simulink model "sim_kalman03_p_u"  (R2015a)
settings: Solver=ode45  StartTime=1  StopTime=100  MaxStep=1  MinStep=1  RelTol=1e-8
undefined symbols (not defined in the file or in its folder): Discrete, Time
libraries: ctrlSharedLib x1
settings Model: Creator=liuqi  LastModifiedBy=liuqi
settings SolverCC: InitialStep=1

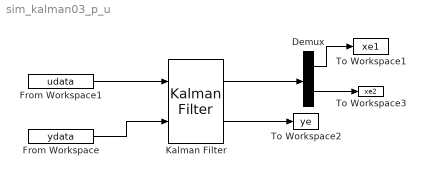
== system sim_kalman03_p_u ==
  Demux : Demux  Outputs=2
  From Workspace : FromWorkspace  VariableName=ydata  SampleTime=1  Interpolate=off  OutputAfterFinalValue=Setting to zero
  From Workspace1 : FromWorkspace  VariableName=udata  SampleTime=1  Interpolate=off  OutputAfterFinalValue=Setting to zero
  Kalman Filter : ctrlSharedLib/Kalman Filter  TimeDomain=Discrete-Time  UseCurrentEstimator=on  ModelSource=Individual A, B, C, D matrices  ModelSourceVariable=sys  A=[1,1;0,1]  B=[0.5;1]  C=[1, 0]  D=0  NumberOfStates=2  NumberOfInputs=2  NumberOfOutputs=2  InitialEstimateSource=Dialog  X0=[10; 0]  P0=10  UseK=off  UseGH=off  NumberOfProcessNoiseInputs=2  G=[0.5, 0, 0; 0, 0.01, 0; 0, 0, 0.001]  TimeInvariantG=on  H=[1, 0,0; 1, 0,0]  TimeInvariantH=on  Q=[0.5, 0; 0, 0.1]  TimeInvariantQ=on  R=25  TimeInvariantR=on  N=0  TimeInvariantN=on  AddInputPort=on  AddEnablePort=off  OutputEstimatedY=on  OutputP=off  Ts=1
  To Workspace1 : ToWorkspace  VariableName=xe1  SaveFormat=Structure With Time  SampleTime=-1
  To Workspace2 : ToWorkspace  VariableName=ye  SaveFormat=Structure With Time  SampleTime=-1
  To Workspace3 : ToWorkspace  VariableName=xe2  SaveFormat=Structure With Time  SampleTime=-1
  wires:
  From Workspace/1 -> Kalman Filter/2
  From Workspace1/1 -> Kalman Filter/1
  Kalman Filter/2 -> To Workspace2/1
  Kalman Filter/1 -> Demux/1
  Demux/1 -> To Workspace1/1
  Demux/2 -> To Workspace3/1
